simulink model "massignment8"  (Simulink 6.0)
settings: Solver=FixedStepDiscrete  StartTime=0.0  StopTime=10.0  RelTol=1e-3
settings Model: Creator=awarlock  LastModifiedBy=awarlock  ExtModeAutoUpdateStatusClock=off
settings OptimizationCC: InlineParams=on

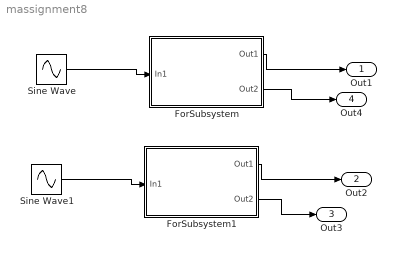
== system massignment8 ==
  ForSubsystem : Subsystem
  ForSubsystem1 : Subsystem
  Sine Wave : Sin  Amplitude=3:7  SampleTime=0.1
  Sine Wave1 : Sin  Amplitude=3:7  SampleTime=0.1
  Out1 : Outport
  Out2 : Outport  Port=2
  Out3 : Outport  Port=3
  Out4 : Outport  Port=4
  wires:
  Sine Wave/1 -> ForSubsystem/1(In1)
  ForSubsystem/1(Out1) -> Out1/1
  Sine Wave1/1 -> ForSubsystem1/1(In1)
  ForSubsystem1/1(Out1) -> Out2/1
  ForSubsystem1/2(Out2) -> Out3/1
  ForSubsystem/2(Out2) -> Out4/1

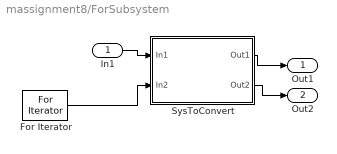
== system massignment8/ForSubsystem ==
  In1 : Inport  Port=1  LatchInput=off
  For Iterator : ForIterator  IterationVariableDataType=double
  SysToConvert : Subsystem  TreatAsAtomicUnit=on
  Out1 : Outport
  Out2 : Outport  Port=2
  wires:
  In1/1 -> SysToConvert/1(In1)
  SysToConvert/1(Out1) -> Out1/1
  For Iterator/1 -> SysToConvert/2(In2)
  SysToConvert/2(Out2) -> Out2/1

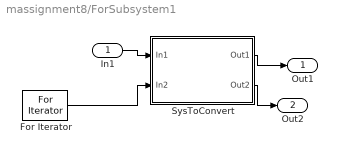
== system massignment8/ForSubsystem1 ==
  In1 : Inport  Port=1  LatchInput=off
  For Iterator : ForIterator  IterationVariableDataType=double
  SysToConvert : Subsystem  TreatAsAtomicUnit=on
  Out1 : Outport
  Out2 : Outport  Port=2
  wires:
  For Iterator/1 -> SysToConvert/2(In2)
  SysToConvert/1(Out1) -> Out1/1
  In1/1 -> SysToConvert/1(In1)
  SysToConvert/2(Out2) -> Out2/1

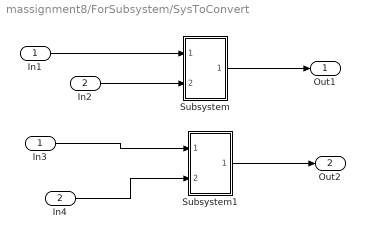
== system massignment8/ForSubsystem/SysToConvert ==
  In1 : Inport  Port=1  LatchInput=off
  In2 : Inport  Port=2  LatchInput=off
  In3 : InportShadow  Port=1  LatchInput=off
  In4 : InportShadow  Port=2  LatchInput=off
  Subsystem : Subsystem  TreatAsAtomicUnit=on
  Subsystem1 : Subsystem  TreatAsAtomicUnit=on
  Out1 : Outport
  Out2 : Outport  Port=2
  wires:
  In1/1 -> Subsystem/1(In1)
  Subsystem/1(Out1) -> Out1/1
  In2/1 -> Subsystem/2(In2)
  Subsystem1/1(Out1) -> Out2/1
  In3/1 -> Subsystem1/1(In1)
  In4/1 -> Subsystem1/2(In2)

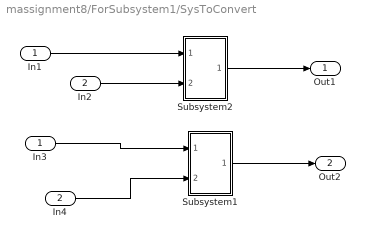
== system massignment8/ForSubsystem1/SysToConvert ==
  In1 : Inport  Port=1  LatchInput=off
  In2 : Inport  Port=2  LatchInput=off
  In3 : InportShadow  Port=1  LatchInput=off
  In4 : InportShadow  Port=2  LatchInput=off
  Subsystem1 : Subsystem  TreatAsAtomicUnit=on
  Subsystem2 : Subsystem  TreatAsAtomicUnit=on
  Out1 : Outport
  Out2 : Outport  Port=2
  wires:
  In4/1 -> Subsystem1/2(In2)
  In3/1 -> Subsystem1/1(In1)
  Subsystem1/1(Out1) -> Out2/1
  In2/1 -> Subsystem2/2(In2)
  Subsystem2/1(Out1) -> Out1/1
  In1/1 -> Subsystem2/1(In1)

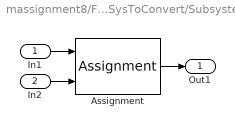
== system massignment8/ForSubsystem/SysToConvert/Subsystem ==
  In1 : Inport  Port=1  LatchInput=off
  In2 : Inport  Port=2  LatchInput=off
  Assignment : Assignment
  Out1 : Outport
  wires:
  In1/1 -> Assignment/1
  Assignment/1 -> Out1/1
  In2/1 -> Assignment/2

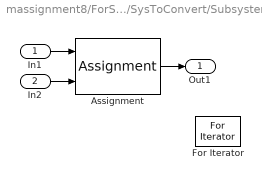
== system massignment8/ForSubsystem/SysToConvert/Subsystem1 ==
  In1 : Inport  Port=1  LatchInput=off
  In2 : Inport  Port=2  LatchInput=off
  Assignment : Assignment
  For Iterator : ForIterator  ShowIterationPort=off  IterationVariableDataType=double
  Out1 : Outport
  wires:
  In2/1 -> Assignment/2
  Assignment/1 -> Out1/1
  In1/1 -> Assignment/1

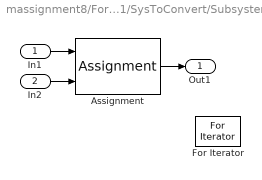
== system massignment8/ForSubsystem1/SysToConvert/Subsystem1 ==
  In1 : Inport  Port=1  LatchInput=off
  In2 : Inport  Port=2  LatchInput=off
  Assignment : Assignment
  For Iterator : ForIterator  ShowIterationPort=off  IterationVariableDataType=double
  Out1 : Outport
  wires:
  In1/1 -> Assignment/1
  Assignment/1 -> Out1/1
  In2/1 -> Assignment/2

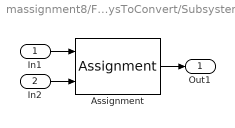
== system massignment8/ForSubsystem1/SysToConvert/Subsystem2 ==
  In1 : Inport  Port=1  LatchInput=off
  In2 : Inport  Port=2  LatchInput=off
  Assignment : Assignment
  Out1 : Outport
  wires:
  In2/1 -> Assignment/2
  Assignment/1 -> Out1/1
  In1/1 -> Assignment/1
